simulink model "PMSM_State_Space_Model"  (R2015b)
settings: Solver=VariableStepAuto  StartTime=0.0  StopTime=10  RelTol=1e-3
values from neighbouring files (symbols this model uses):
  c_drag_pro = c_drag*G1.^3*r.^3/G2.^3    [Control_Parameters.m]    (also in M_fil_til_jacob.m; PMSM_State_Space_Parameters.m)
  J_pro = (m*r^2+J_G2)*(G1/G2)^2 + J_G1    (= 0.281547798877)    [Control_Parameters.m]    (also in M_fil_til_jacob.m; PMSM_State_Space_Parameters.m)
  Kt = .07329    (= 0.07329)    [Control_Parameters.m]    (also in M_fil_til_jacob.m; PMSM_State_Space_Parameters.m)
  R = .013/2    (= 0.0065)    [Control_Parameters.m]    (also in M_fil_til_jacob.m; PMSM_State_Space_Parameters.m)
  TS = L/R    (= 0.00615384615385)    [Control_Parameters.m]    (also in M_fil_til_jacob.m; PMSM_State_Space_Parameters.m)
settings Model: Creator=Morten  LastModifiedBy=Morten

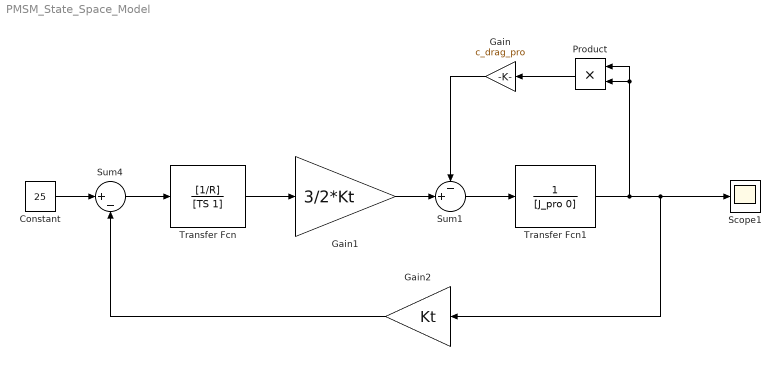
== system PMSM_State_Space_Model ==
  Constant : Constant  Value=25
  Gain : Gain  Gain=c_drag_pro
  Gain1 : Gain  Gain=3/2*Kt
  Gain2 : Gain  Gain=Kt
  Product : Product
  Scope1 : Scope
  Sum1 : Sum  Inputs=-+|
  Sum4 : Sum  Inputs=|+-
  Transfer Fcn : TransferFcn  Numerator=[1/R]  Denominator=[TS 1]
  Transfer Fcn1 : TransferFcn  Denominator=[J_pro 0]
  wires:
  Constant/1 -> Sum4/1
  Gain2/1 -> Sum4/2
  Sum4/1 -> Transfer Fcn/1
  Transfer Fcn/1 -> Gain1/1
  Gain/1 -> Sum1/1
  Transfer Fcn1/1 -> Gain2/1, Scope1/1, Product/1, Product/2
  Sum1/1 -> Transfer Fcn1/1
  Gain1/1 -> Sum1/2
  Product/1 -> Gain/1
